simulink model "Test_of_StateFeedbackCtrl_CP_Controller"  (R2023a)
settings: Solver=ode8  StartTime=0.0  StopTime=150  FixedStep=0.001  RelTol=1e-3
libraries: simulink x4
settings Model: Creator=邓宇飞  LastModifiedBy=邓宇飞

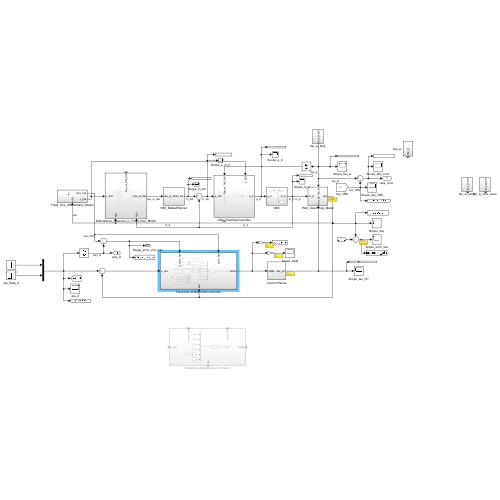
[thumbnail: Simulink's stored preview of the top-level diagram]
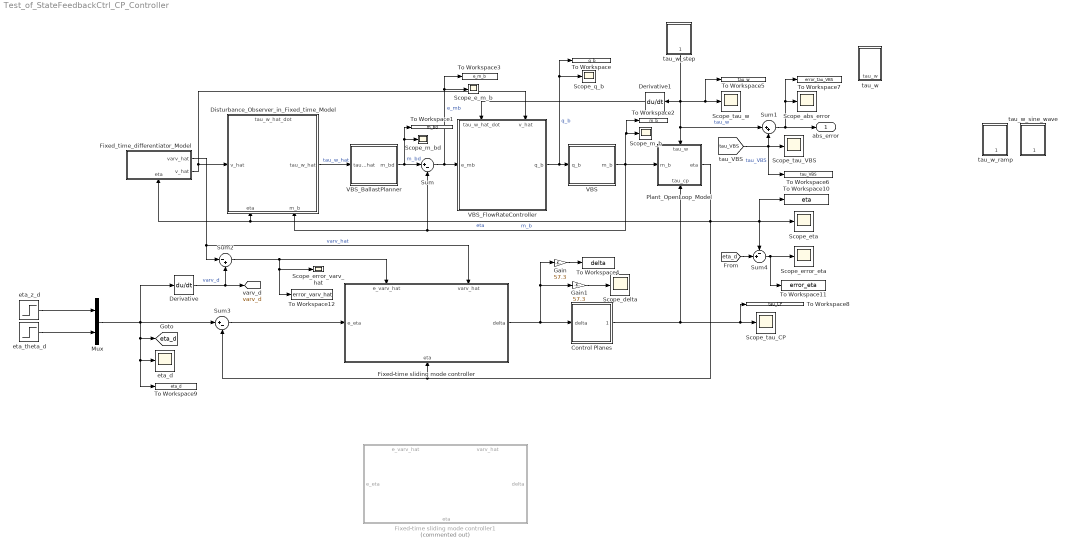
== system Test_of_StateFeedbackCtrl_CP_Controller ==
  Control Planes : Subsystem
  Derivative : Derivative
  Derivative1 : Derivative
  Disturbance_Observer_in_Fixed_time_Model : Subsystem
      settings: PortSchema="{\"entries\":[{\"content\":{\"sides\":[{\"content\":{\"connectorIds\":[\"In1\"]},\"type\":\"ConnectorPlacement.EquallySpacedRectSide\",\"uuid\":\"977a3149-1921-48fe-b96a-a4ad28c91371\"},{\"content\":{\"connectorIds\":[\"Out1\"],\"side\":\"RIGHT\"},\"type\":\"ConnectorPlacement.EquallySpacedRectSide\",\"uuid\":\"fff94096-65c1-4681-8bdf-eed371b61c52\"},{\"content\":{\"connectorIds\":[\"Out2\"],\"side\":\"TOP\"},\"type\":\"ConnectorPlacement.EquallySpacedRectSide\",\"uuid\":\"5bed714d-ab4b-433b-a946-feaea2816cb1\"},{\"content\":{\"connectorIds\":[\"In2\",\"In3\"],\"side\":\"BOTTOM\"},\"type\":\"ConnectorPlacement.EquallySpacedRectSide\",\"uuid\":\"4ad85521-d335-4ab1-88b6-9b8c0a3b2785\"}]},\"type\":\"ConnectorPlacement.EquallySpacedConnector\",\"uuid\":\"7c33b186-f768-465e-b799-f94ef9fdf411\"}],\"packageUris\":[\"http://schema.mathworks.com/mf0/Connector/R2020b\"],\"version\":\"1.0\"}"
  Fixed-time sliding mode controller : Subsystem
      settings: PortSchema="{\"entries\":[{\"content\":{\"sides\":[{\"content\":{\"connectorIds\":[\"In1\"]},\"type\":\"ConnectorPlacement.EquallySpacedRectSide\",\"uuid\":\"f7eec32a-11e5-493e-91a4-aa23e7798835\"},{\"content\":{\"connectorIds\":[\"Out1\"],\"side\":\"RIGHT\"},\"type\":\"ConnectorPlacement.EquallySpacedRectSide\",\"uuid\":\"2b78eec5-73c8-4d02-9319-0fb2d1bcee33\"},{\"content\":{\"connectorIds\":[\"In2\",\"In3\"],\"side\":\"TOP\"},\"type\":\"ConnectorPlacement.EquallySpacedRectSide\",\"uuid\":\"6bb67a89-6549-4a25-872d-286d7aa8440b\"},{\"content\":{\"connectorIds\":[\"In4\"],\"side\":\"BOTTOM\"},\"type\":\"ConnectorPlacement.EquallySpacedRectSide\",\"uuid\":\"a7c480fa-a393-4283-926e-8262b2c36ba1\"}]},\"type\":\"ConnectorPlacement.EquallySpacedConnector\",\"uuid\":\"ac88fafb-ad61-4f2d-a744-8be38b32af3c\"}],\"packageUris\":[\"http://schema.mathworks.com/mf0/Connector/R2020b\"],\"version\":\"1.0\"}"
  Fixed-time sliding mode controller1 : Subsystem  Commented=on
      settings: PortSchema="{\"entries\":[{\"content\":{\"sides\":[{\"content\":{\"connectorIds\":[\"In1\"]},\"type\":\"ConnectorPlacement.EquallySpacedRectSide\",\"uuid\":\"f7eec32a-11e5-493e-91a4-aa23e7798835\"},{\"content\":{\"connectorIds\":[\"Out1\"],\"side\":\"RIGHT\"},\"type\":\"ConnectorPlacement.EquallySpacedRectSide\",\"uuid\":\"2b78eec5-73c8-4d02-9319-0fb2d1bcee33\"},{\"content\":{\"connectorIds\":[\"In2\",\"In3\"],\"side\":\"TOP\"},\"type\":\"ConnectorPlacement.EquallySpacedRectSide\",\"uuid\":\"6bb67a89-6549-4a25-872d-286d7aa8440b\"},{\"content\":{\"connectorIds\":[\"In4\"],\"side\":\"BOTTOM\"},\"type\":\"ConnectorPlacement.EquallySpacedRectSide\",\"uuid\":\"a7c480fa-a393-4283-926e-8262b2c36ba1\"}]},\"type\":\"ConnectorPlacement.EquallySpacedConnector\",\"uuid\":\"ac88fafb-ad61-4f2d-a744-8be38b32af3c\"}],\"packageUris\":[\"http://schema.mathworks.com/mf0/Connector/R2020b\"],\"version\":\"1.0\"}"
  Fixed_time_differentiator_Model : Subsystem
      settings: PortSchema="{\"entries\":[{\"content\":{\"sides\":[{\"content\":{},\"type\":\"ConnectorPlacement.EquallySpacedRectSide\",\"uuid\":\"509b689f-cae1-4523-9372-2499bd3b7d9d\"},{\"content\":{\"connectorIds\":[\"Out1\",\"Out2\"],\"side\":\"RIGHT\"},\"type\":\"ConnectorPlacement.EquallySpacedRectSide\",\"uuid\":\"a1df743b-e6a9-4451-86f2-27990c18dc24\"},{\"content\":{\"side\":\"TOP\"},\"type\":\"ConnectorPlacement.EquallySpacedRectSide\",\"uuid\":\"5149f091-ad88-4d80-a39f-36dd9d24fd7a\"},{\"content\":{\"connectorIds\":[\"In1\"],\"side\":\"BOTTOM\"},\"type\":\"ConnectorPlacement.EquallySpacedRectSide\",\"uuid\":\"b5eefe9f-7883-4d8e-a8af-dce689347657\"}]},\"type\":\"ConnectorPlacement.EquallySpacedConnector\",\"uuid\":\"61175d6f-7ec4-4947-9258-193f13282eb9\"}],\"packageUris\":[\"http://schema.mathworks.com/mf0/Connector/R2020b\"],\"version\":\"1.0\"}"
  Gain : Gain  Gain=57.3
  Gain1 : Gain  Gain=57.3
  Mux : Mux  Inputs=2
  Plant_OpenLoop_Model : Subsystem
      settings: PortSchema="{\"entries\":[{\"content\":{\"sides\":[{\"content\":{\"connectorIds\":[\"In1\"]},\"type\":\"ConnectorPlacement.EquallySpacedRectSide\",\"uuid\":\"171ab365-2c9c-477f-ab94-6e1b535ce398\"},{\"content\":{\"connectorIds\":[\"Out1\"],\"side\":\"RIGHT\"},\"type\":\"ConnectorPlacement.EquallySpacedRectSide\",\"uuid\":\"68d15153-0085-4baf-9515-c294b6b9b8eb\"},{\"content\":{\"connectorIds\":[\"In2\"],\"side\":\"TOP\"},\"type\":\"ConnectorPlacement.EquallySpacedRectSide\",\"uuid\":\"3f887e7e-8b06-4bf2-b39d-d49324deef58\"},{\"content\":{\"connectorIds\":[\"In3\"],\"side\":\"BOTTOM\"},\"type\":\"ConnectorPlacement.EquallySpacedRectSide\",\"uuid\":\"0c56d0aa-527a-42c0-aa98-8ee52c9400f1\"}]},\"type\":\"ConnectorPlacement.EquallySpacedConnector\",\"uuid\":\"a8f2799e-4d6b-4adf-9803-c3f607cd4a91\"}],\"packageUris\":[\"http://schema.mathworks.com/mf0/Connector/R2020b\"],\"version\":\"1.0\"}"
  Scope_abs_error : Scope
  Scope_delta : Scope
  Scope_e_m_b : Scope
  Scope_error_eta : Scope
  Scope_error_varv_hat : Scope
  Scope_eta : Scope
  Scope_m_b : Scope
  Scope_m_bd : Scope
  Scope_q_b : Scope
  Scope_tau_CP : Scope
  Scope_tau_VBS : Scope
  Scope_tau_w : Scope
  Sum : Sum  Inputs=|+-
  Sum1 : Sum  Inputs=|++
  Sum2 : Sum  Inputs=|-+
  Sum3 : Sum  Inputs=|+-
  Sum4 : Sum  Inputs=-+|
  To Workspace : ToWorkspace  VariableName=q_b  SaveFormat=Timeseries  SampleTime=-1
  To Workspace1 : ToWorkspace  VariableName=m_bd  SaveFormat=Timeseries  SampleTime=-1
  To Workspace10 : ToWorkspace  VariableName=eta  SaveFormat=Timeseries  SampleTime=-1
  To Workspace11 : ToWorkspace  VariableName=error_eta  SaveFormat=Timeseries  SampleTime=-1
  To Workspace12 : ToWorkspace  VariableName=error_varv_hat  SaveFormat=Timeseries  SampleTime=-1
  To Workspace2 : ToWorkspace  VariableName=m_b  SaveFormat=Timeseries  SampleTime=-1
  To Workspace3 : ToWorkspace  VariableName=e_m_b  SaveFormat=Timeseries  SampleTime=-1
  To Workspace4 : ToWorkspace  VariableName=delta  SaveFormat=Timeseries  SampleTime=-1
  To Workspace5 : ToWorkspace  VariableName=tau_w  SaveFormat=Timeseries  SampleTime=-1
  To Workspace6 : ToWorkspace  VariableName=tau_VBS  SaveFormat=Timeseries  SampleTime=-1
  To Workspace7 : ToWorkspace  VariableName=error_tau_VBS  SaveFormat=Timeseries  SampleTime=-1
  To Workspace8 : ToWorkspace  VariableName=tau_CP  SaveFormat=Timeseries  SampleTime=-1
  To Workspace9 : ToWorkspace  VariableName=eta_d  SaveFormat=Timeseries  SampleTime=-1
  VBS : Subsystem
  VBS_BallastPlanner : Subsystem
  VBS_FlowRateController : Subsystem
      settings: PortSchema="{\"entries\":[{\"content\":{\"sides\":[{\"content\":{\"connectorIds\":[\"In1\"]},\"type\":\"ConnectorPlacement.EquallySpacedRectSide\",\"uuid\":\"977a3149-1921-48fe-b96a-a4ad28c91371\"},{\"content\":{\"connectorIds\":[\"Out1\"],\"side\":\"RIGHT\"},\"type\":\"ConnectorPlacement.EquallySpacedRectSide\",\"uuid\":\"fff94096-65c1-4681-8bdf-eed371b61c52\"},{\"content\":{\"connectorIds\":[\"In2\",\"In3\"],\"side\":\"TOP\"},\"type\":\"ConnectorPlacement.EquallySpacedRectSide\",\"uuid\":\"5bed714d-ab4b-433b-a946-feaea2816cb1\"}]},\"type\":\"ConnectorPlacement.EquallySpacedConnector\",\"uuid\":\"7c33b186-f768-465e-b799-f94ef9fdf411\"}],\"packageUris\":[\"http://schema.mathworks.com/mf0/Connector/R2020b\"],\"version\":\"1.0\"}"
  eta_d : Scope
  eta_theta_d : Step  Time=0  After=0  SampleTime=0
  eta_z_d : Step  Time=0  Before=1  SampleTime=0
  tau_w : Subsystem
  tau_w_ramp : Subsystem
      settings: PortSchema="{\"entries\":[{\"content\":{\"sides\":[{\"content\":{},\"type\":\"ConnectorPlacement.EquallySpacedRectSide\",\"uuid\":\"4f4de30a-0d0b-4bec-80d6-0206e412bf93\"},{\"content\":{\"side\":\"RIGHT\"},\"type\":\"ConnectorPlacement.EquallySpacedRectSide\",\"uuid\":\"99f054dc-7a49-4f3a-aacd-86d3d985c053\"},{\"content\":{\"side\":\"TOP\"},\"type\":\"ConnectorPlacement.EquallySpacedRectSide\",\"uuid\":\"fb1c8c59-da3b-46d1-8a85-15943150b176\"},{\"content\":{\"connectorIds\":[\"Out1\"],\"side\":\"BOTTOM\"},\"type\":\"ConnectorPlacement.EquallySpacedRectSide\",\"uuid\":\"0ca0dd3c-9837-4edc-a372-abf376ee5c7a\"}]},\"type\":\"ConnectorPlacement.EquallySpacedConnector\",\"uuid\":\"b18296a3-8797-45d2-90ea-b6dd47f9d7d0\"}],\"packageUris\":[\"http://schema.mathworks.com/mf0/Connector/R2020b\"],\"version\":\"1.0\"}"
  tau_w_sine_wave : Subsystem
      settings: PortSchema="{\"entries\":[{\"content\":{\"sides\":[{\"content\":{},\"type\":\"ConnectorPlacement.EquallySpacedRectSide\",\"uuid\":\"4f4de30a-0d0b-4bec-80d6-0206e412bf93\"},{\"content\":{\"side\":\"RIGHT\"},\"type\":\"ConnectorPlacement.EquallySpacedRectSide\",\"uuid\":\"99f054dc-7a49-4f3a-aacd-86d3d985c053\"},{\"content\":{\"side\":\"TOP\"},\"type\":\"ConnectorPlacement.EquallySpacedRectSide\",\"uuid\":\"fb1c8c59-da3b-46d1-8a85-15943150b176\"},{\"content\":{\"connectorIds\":[\"Out1\"],\"side\":\"BOTTOM\"},\"type\":\"ConnectorPlacement.EquallySpacedRectSide\",\"uuid\":\"20ef5005-9f22-4516-b524-19691bb7c6fc\"}]},\"type\":\"ConnectorPlacement.EquallySpacedConnector\",\"uuid\":\"b18296a3-8797-45d2-90ea-b6dd47f9d7d0\"}],\"packageUris\":[\"http://schema.mathworks.com/mf0/Connector/R2020b\"],\"version\":\"1.0\"}"
  tau_w_step : Subsystem
      settings: PortSchema="{\"entries\":[{\"content\":{\"sides\":[{\"content\":{},\"type\":\"ConnectorPlacement.EquallySpacedRectSide\",\"uuid\":\"4f4de30a-0d0b-4bec-80d6-0206e412bf93\"},{\"content\":{\"side\":\"RIGHT\"},\"type\":\"ConnectorPlacement.EquallySpacedRectSide\",\"uuid\":\"99f054dc-7a49-4f3a-aacd-86d3d985c053\"},{\"content\":{\"side\":\"TOP\"},\"type\":\"ConnectorPlacement.EquallySpacedRectSide\",\"uuid\":\"fb1c8c59-da3b-46d1-8a85-15943150b176\"},{\"content\":{\"connectorIds\":[\"Out1\"],\"side\":\"BOTTOM\"},\"type\":\"ConnectorPlacement.EquallySpacedRectSide\",\"uuid\":\"1bc79977-bf79-43c9-a15f-49778b641523\"}]},\"type\":\"ConnectorPlacement.EquallySpacedConnector\",\"uuid\":\"b18296a3-8797-45d2-90ea-b6dd47f9d7d0\"}],\"packageUris\":[\"http://schema.mathworks.com/mf0/Connector/R2020b\"],\"version\":\"1.0\"}"
  abs_error : Outport
  tag scope: eta_d=global, varv_d=global
  wires:
  Fixed-time sliding mode controller/1(delta) -> Gain/1, Gain1/1, Control Planes/1(delta)
  Disturbance_Observer_in_Fixed_time_Model/1(tau_w_hat) -> VBS_BallastPlanner/1(tau_w_hat)  "tau_w_hat"
  VBS_FlowRateController/1(q_b) -> To Workspace/1, Scope_q_b/1, VBS/1(q_b)  "q_b"
  [tau_VBS] -> To Workspace6/1, Scope_tau_VBS/1, Sum1/2  "tau_VBS"
  VBS/1(m_b) -> To Workspace2/1, Scope_m_b/1, Disturbance_Observer_in_Fixed_time_Model/3(m_b), Sum/2, Plant_OpenLoop_Model/1(m_b)  "m_b"
  Plant_OpenLoop_Model/1(eta) -> To Workspace10/1, Sum4/1, Scope_eta/1, Sum3/2, Fixed-time sliding mode controller/4(eta), Fixed_time_differentiator_Model/1(eta), Disturbance_Observer_in_Fixed_time_Model/2(eta)  "eta"
  Sum1/1 -> To Workspace7/1, Scope_abs_error/1, abs_error/1
  tau_w_step/1(tau_w_step) -> Derivative1/1, Plant_OpenLoop_Model/2(tau_w), Sum1/1, To Workspace5/1, Scope_tau_w/1  "tau_w"
  Fixed_time_differentiator_Model/1(varv_hat) -> Fixed-time sliding mode controller/3(varv_hat), Sum2/1  "varv_hat"
  Sum/1 -> VBS_FlowRateController/1(e_mb), To Workspace3/1, Scope_e_m_b/1  "e_mb"
  VBS_BallastPlanner/1(m_bd) -> Sum/1, To Workspace1/1, Scope_m_bd/1  "m_bd"
  Mux/1 -> To Workspace9/1, eta_d/1, [eta_d], Derivative/1, Sum3/1
  Derivative/1 -> [varv_d], Sum2/2  "varv_d"
  Sum2/1 -> Fixed-time sliding mode controller/2(e_varv_hat), To Workspace12/1, Scope_error_varv_hat/1
  Sum3/1 -> Fixed-time sliding mode controller/1(e_eta)
  eta_z_d/1 -> Mux/1
  eta_theta_d/1 -> Mux/2
  Fixed_time_differentiator_Model/2(v_hat) -> Disturbance_Observer_in_Fixed_time_Model/1(v_hat), VBS_FlowRateController/3(v_hat)
  Gain/1 -> To Workspace4/1
  Gain1/1 -> Scope_delta/1
  [eta_d] -> Sum4/2
  Sum4/1 -> To Workspace11/1, Scope_error_eta/1
  Derivative1/1 -> VBS_FlowRateController/2(tau_w_hat_dot)
  Control Planes/1(tau_cp) -> To Workspace8/1, Scope_tau_CP/1, Plant_OpenLoop_Model/3(tau_cp)

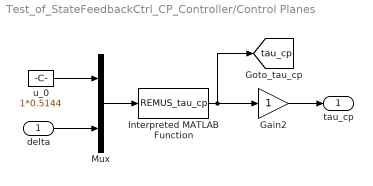
== system Test_of_StateFeedbackCtrl_CP_Controller/Control Planes ==
  delta : Inport
  Gain2 : Gain
  Interpreted MATLAB Function : MATLABFcn  MATLABFcn=REMUS_tau_cp
  Mux : Mux  Inputs=2
  u_0 : Constant  Value=1*0.5144
  tau_cp : Outport
  tag scope: tau_cp=global
  wires:
  delta/1 -> Mux/2
  u_0/1 -> Mux/1
  Mux/1 -> Interpreted MATLAB Function/1
  Interpreted MATLAB Function/1 -> Gain2/1, [tau_cp]
  Gain2/1 -> tau_cp/1

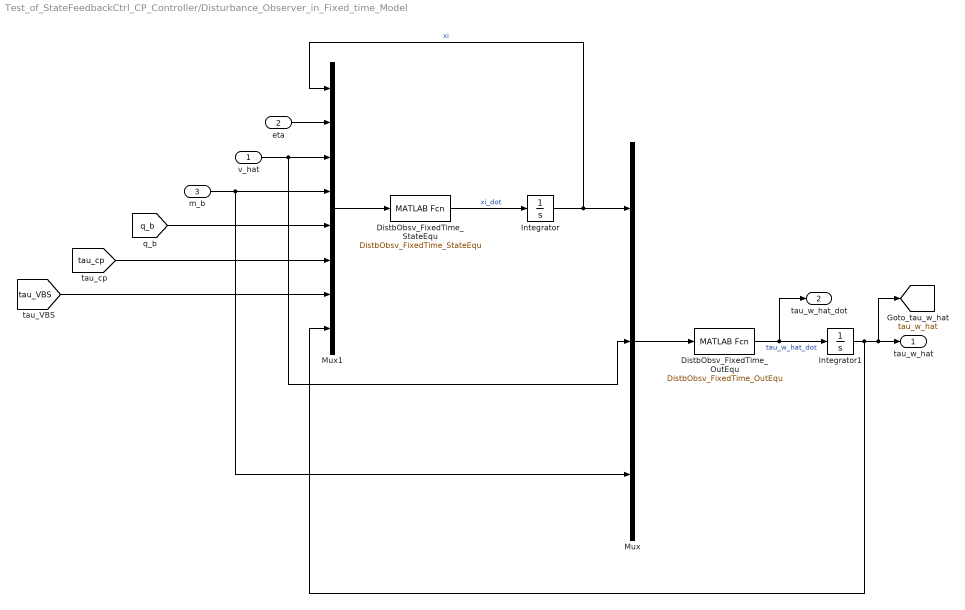
== system Test_of_StateFeedbackCtrl_CP_Controller/Disturbance_Observer_in_Fixed_time_Model ==
  v_hat : Inport
  eta : Inport  Port=2
  m_b : Inport  Port=3
  DistbObsv_FixedTime_OutEqu : MATLABFcn  MATLABFcn=DistbObsv_FixedTime_OutEqu  OutputDimensions=2  OutputSignalType=real
  DistbObsv_FixedTime_StateEqu : MATLABFcn  MATLABFcn=DistbObsv_FixedTime_StateEqu  OutputDimensions=2  OutputSignalType=real
  Integrator : Integrator
  Integrator1 : Integrator
  Mux : Mux  Inputs=3
  Mux1 : Mux  Inputs=8
  tau_w_hat : Outport
  tau_w_hat_dot : Outport  Port=2
  tag scope: tau_w_hat=global
  wires:
  Integrator1/1 -> [tau_w_hat], tau_w_hat/1, Mux1/8
  Integrator/1 -> Mux1/1, Mux/1  "xi"
  DistbObsv_FixedTime_OutEqu/1 -> tau_w_hat_dot/1, Integrator1/1  "tau_w_hat_dot"
  Mux/1 -> DistbObsv_FixedTime_OutEqu/1
  Mux1/1 -> DistbObsv_FixedTime_StateEqu/1
  DistbObsv_FixedTime_StateEqu/1 -> Integrator/1  "xi_dot"
  eta/1 -> Mux1/2
  v_hat/1 -> Mux/2, Mux1/3
  m_b/1 -> Mux/3, Mux1/4
  [q_b] -> Mux1/5
  [tau_cp] -> Mux1/6
  [tau_VBS] -> Mux1/7

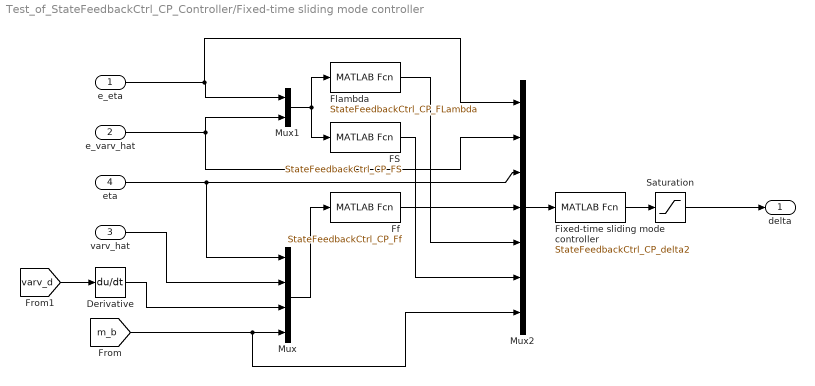
== system Test_of_StateFeedbackCtrl_CP_Controller/Fixed-time sliding mode controller ==
  e_eta : Inport
  e_varv_hat : Inport  Port=2
  varv_hat : Inport  Port=3
  eta : Inport  Port=4
  Derivative : Derivative
  FS : MATLABFcn  MATLABFcn=StateFeedbackCtrl_CP_FS  OutputDimensions=2  OutputSignalType=real
  Ff : MATLABFcn  MATLABFcn=StateFeedbackCtrl_CP_Ff  OutputDimensions=2  OutputSignalType=real
  Fixed-time sliding mode controller : MATLABFcn  MATLABFcn=StateFeedbackCtrl_CP_delta2  OutputDimensions=2  OutputSignalType=real
  Flambda : MATLABFcn  MATLABFcn=StateFeedbackCtrl_CP_FLambda  OutputDimensions=2  OutputSignalType=real
  Mux : Mux
  Mux1 : Mux  Inputs=2
  Mux2 : Mux  Inputs=7
  Saturation : Saturate  UpperLimit=pi/6  LowerLimit=-pi/6
  delta : Outport
  wires:
  eta/1 -> Mux2/3, Mux/1
  Derivative/1 -> Mux/3
  varv_hat/1 -> Mux/2
  e_eta/1 -> Mux2/1, Mux1/1
  e_varv_hat/1 -> Mux1/2, Mux2/2
  Fixed-time sliding mode controller/1 -> Saturation/1
  [varv_d] -> Derivative/1
  Mux/1 -> Ff/1
  [m_b] -> Mux2/7, Mux/4
  Mux1/1 -> Flambda/1, FS/1
  Ff/1 -> Mux2/4
  Flambda/1 -> Mux2/5
  FS/1 -> Mux2/6
  Mux2/1 -> Fixed-time sliding mode controller/1
  Saturation/1 -> delta/1

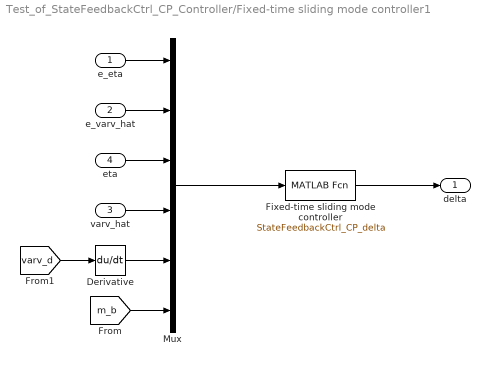
== system Test_of_StateFeedbackCtrl_CP_Controller/Fixed-time sliding mode controller1 ==
  e_eta : Inport
  e_varv_hat : Inport  Port=2
  varv_hat : Inport  Port=3
  eta : Inport  Port=4
  Derivative : Derivative
  Fixed-time sliding mode controller : MATLABFcn  MATLABFcn=StateFeedbackCtrl_CP_delta  OutputDimensions=2  OutputSignalType=real
  Mux : Mux  Inputs=6
  delta : Outport
  wires:
  eta/1 -> Mux/3
  Derivative/1 -> Mux/5
  varv_hat/1 -> Mux/4
  [m_b] -> Mux/6
  e_eta/1 -> Mux/1
  Mux/1 -> Fixed-time sliding mode controller/1
  e_varv_hat/1 -> Mux/2
  Fixed-time sliding mode controller/1 -> delta/1
  [varv_d] -> Derivative/1

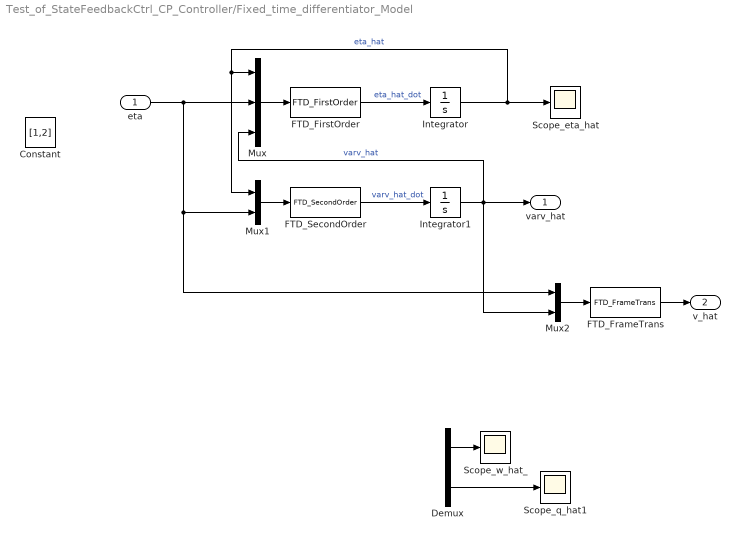
== system Test_of_StateFeedbackCtrl_CP_Controller/Fixed_time_differentiator_Model ==
  eta : Inport
  Constant : Constant  Value=[1,2]
  Demux : Demux  Outputs=2
  FTD_FirstOrder : MATLABFcn  MATLABFcn=FTD_FirstOrder  OutputDimensions=2
  FTD_FrameTrans : MATLABFcn  MATLABFcn=FTD_FrameTrans
  FTD_SecondOrder : MATLABFcn  MATLABFcn=FTD_SecondOrder  OutputDimensions=2
  Integrator : Integrator
  Integrator1 : Integrator
  Mux : Mux  Inputs=3
  Mux1 : Mux  Inputs=2
  Mux2 : Mux  Inputs=2
  Scope_eta_hat : Scope
  Scope_q_hat1 : Scope
  Scope_w_hat_ : Scope
  varv_hat : Outport
  v_hat : Outport  Port=2
  wires:
  Demux/1 -> Scope_w_hat_/1
  Integrator/1 -> Mux1/1, Mux/1, Scope_eta_hat/1  "eta_hat"
  Integrator1/1 -> Mux2/2, varv_hat/1, Mux/3  "varv_hat"
  Mux/1 -> FTD_FirstOrder/1
  Mux1/1 -> FTD_SecondOrder/1
  Demux/2 -> Scope_q_hat1/1
  FTD_SecondOrder/1 -> Integrator1/1  "varv_hat_dot"
  FTD_FirstOrder/1 -> Integrator/1  "eta_hat_dot"
  FTD_FrameTrans/1 -> v_hat/1
  Mux2/1 -> FTD_FrameTrans/1
  eta/1 -> Mux2/1, Mux1/2, Mux/2

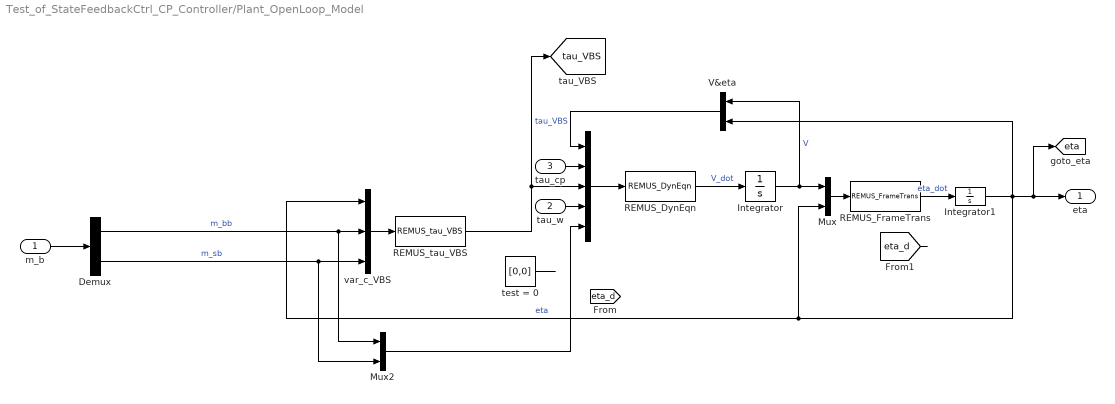
== system Test_of_StateFeedbackCtrl_CP_Controller/Plant_OpenLoop_Model ==
  m_b : Inport
  tau_w : Inport  Port=2
  tau_cp : Inport  Port=3
  " " : Mux  Inputs=5
  Demux : Demux  Outputs=2
  Integrator : Integrator
  Integrator1 : Integrator  InitialCondition=[0;0]
  Mux : Mux  Inputs=2
  Mux2 : Mux  Inputs=2
  REMUS_DynEqn : MATLABFcn  MATLABFcn=REMUS_DynEqn  OutputDimensions=2
  REMUS_FrameTrans : MATLABFcn  MATLABFcn=REMUS_FrameTrans  OutputDimensions=2
  REMUS_tau_VBS : MATLABFcn  MATLABFcn=REMUS_tau_VBS  OutputDimensions=2
  V&eta : Mux  Inputs=2
  test = 0 : Constant  Value=[0,0]
  var_c_VBS : Mux  Inputs=3
  eta : Outport
  tag scope: eta=global, tau_VBS=global
  wires:
  REMUS_DynEqn/1 -> Integrator/1  "V_dot"
  Integrator1/1 -> Mux/2, var_c_VBS/1, [eta], eta/1, V&eta/2  "eta"
  test = 0/1 -> ?
  Demux/2 -> Mux2/2, var_c_VBS/3  "m_sb"
  Mux/1 -> REMUS_FrameTrans/1
  " "/1 -> REMUS_DynEqn/1
  Integrator/1 -> Mux/1, V&eta/1  "V"
  Demux/1 -> Mux2/1, var_c_VBS/2  "m_bb"
  V&eta/1 -> " "/1
  REMUS_tau_VBS/1 -> [tau_VBS], " "/3  "tau_VBS"
  tau_w/1 -> " "/4
  REMUS_FrameTrans/1 -> Integrator1/1  "eta_dot"
  var_c_VBS/1 -> REMUS_tau_VBS/1
  Mux2/1 -> " "/5
  m_b/1 -> Demux/1
  tau_cp/1 -> " "/2
  [eta_d] -> ?

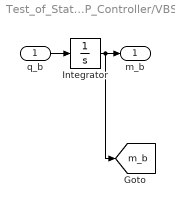
== system Test_of_StateFeedbackCtrl_CP_Controller/VBS ==
  q_b : Inport
  Integrator : Integrator
  m_b : Outport
  tag scope: m_b=global
  wires:
  q_b/1 -> Integrator/1
  Integrator/1 -> [m_b], m_b/1

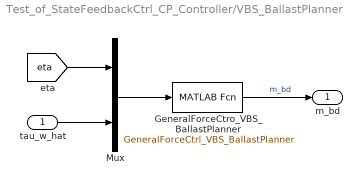
== system Test_of_StateFeedbackCtrl_CP_Controller/VBS_BallastPlanner ==
  tau_w_hat : Inport
  GeneralForceCtro_VBS_BallastPlanner : MATLABFcn  MATLABFcn=GeneralForceCtrl_VBS_BallastPlanner  OutputDimensions=2  OutputSignalType=real
  Mux : Mux  Inputs=2
  m_bd : Outport
  wires:
  Mux/1 -> GeneralForceCtro_VBS_BallastPlanner/1
  GeneralForceCtro_VBS_BallastPlanner/1 -> m_bd/1  "m_bd"
  [eta] -> Mux/1
  tau_w_hat/1 -> Mux/2

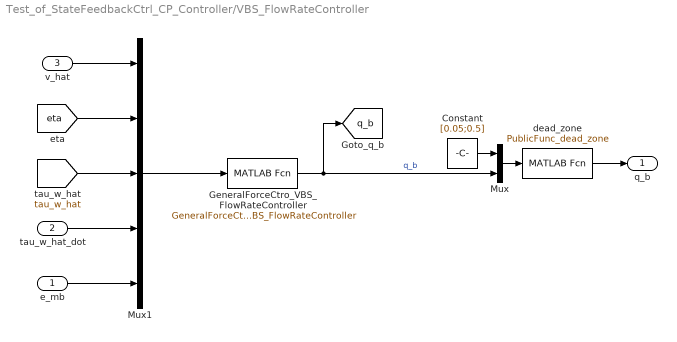
== system Test_of_StateFeedbackCtrl_CP_Controller/VBS_FlowRateController ==
  e_mb : Inport
  tau_w_hat_dot : Inport  Port=2
  v_hat : Inport  Port=3
  Constant : Constant  Value=[0.05;0.5]
  GeneralForceCtro_VBS_FlowRateController : MATLABFcn  MATLABFcn=GeneralForceCtrl_VBS_FlowRateController  OutputDimensions=2  OutputSignalType=real
  Mux : Mux  Inputs=2
  Mux1 : Mux  Inputs=5
  dead_zone : MATLABFcn  MATLABFcn=PublicFunc_dead_zone
  q_b : Outport
  tag scope: q_b=global
  wires:
  Mux1/1 -> GeneralForceCtro_VBS_FlowRateController/1
  GeneralForceCtro_VBS_FlowRateController/1 -> Mux/2, [q_b]  "q_b"
  v_hat/1 -> Mux1/1
  [eta] -> Mux1/2
  [tau_w_hat] -> Mux1/3
  tau_w_hat_dot/1 -> Mux1/4
  e_mb/1 -> Mux1/5
  dead_zone/1 -> q_b/1
  Constant/1 -> Mux/1
  Mux/1 -> dead_zone/1

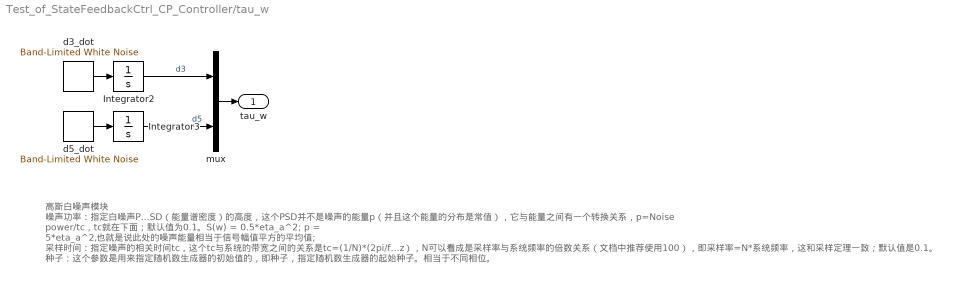
== system Test_of_StateFeedbackCtrl_CP_Controller/tau_w ==
  note: 高斯白噪声模块
      | 噪声功率：指定白噪声PSD（能量谱密度）的高度，这个PSD并不是噪声的能量p（并且这个能量的分布是常值），它与能量之间有一个转换关系，p=Noise power/tc，tc就在下面；默认值为0.1。S(w) = 0.5*eta_a^2;
      | p = 5*eta_a^2;也就是说此处的噪声能量相当于信号幅值平方的平均值;
      | 采样时间：指定噪声的相关时间tc，这个tc与系统的带宽之间的关系是tc=(1/N)*(2pi/fmax)，其中fmax是系统的带宽（实际上是角频率，fmax=2*pi*f，这个f才是我们常使用的频率Hz），N可以看成是采样率与系统频率的倍数关系（文档中推荐使用100），即采样率=N*系统频率，这和采样定理一致；默认值是0.1。
      | 种子：这个参数是用来指定随机数生成器的初始值的，即种子，指定随机数生成器的起始种子。相当于不同相位。
  Integrator2 : Integrator
  Integrator3 : Integrator
  d3_dot : simulink/Sources/Band-Limited White Noise  Cov=[0.5]  Ts=0.1  seed=[2]
  d5_dot : simulink/Sources/Band-Limited White Noise  Cov=[0.1]  Ts=0.1  seed=[3]
  mux : Mux  Inputs=2
  tau_w : Outport
  wires:
  Integrator3/1 -> mux/2  "d5"
  d5_dot/1 -> Integrator3/1
  d3_dot/1 -> Integrator2/1
  mux/1 -> tau_w/1
  Integrator2/1 -> mux/1  "d3"

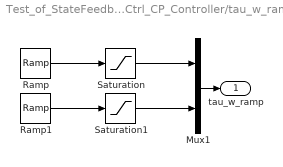
== system Test_of_StateFeedbackCtrl_CP_Controller/tau_w_ramp ==
  Mux1 : Mux  Inputs=2
  Ramp : simulink/Sources/Ramp  slope=1  start=0  InitialOutput=0
  Ramp1 : simulink/Sources/Ramp  slope=1  start=0  InitialOutput=0
  Saturation : Saturate  UpperLimit=10  LowerLimit=0
  Saturation1 : Saturate  UpperLimit=10  LowerLimit=0
  tau_w_ramp : Outport
  wires:
  Mux1/1 -> tau_w_ramp/1
  Ramp/1 -> Saturation/1
  Saturation/1 -> Mux1/1
  Ramp1/1 -> Saturation1/1
  Saturation1/1 -> Mux1/2

== system Test_of_StateFeedbackCtrl_CP_Controller/tau_w_sine_wave ==
  Mux2 : Mux  Inputs=2
  Sine Wave : Sin  Amplitude=15  Frequency=0.1*pi  Phase=0.5*pi  SampleTime=0
  Sine Wave1 : Sin  Amplitude=15  Frequency=0.1*pi  Phase=0.5*pi  SampleTime=0
  tau_w_sine_wave : Outport
  wires:
  Sine Wave1/1 -> Mux2/2
  Sine Wave/1 -> Mux2/1
  Mux2/1 -> tau_w_sine_wave/1

== system Test_of_StateFeedbackCtrl_CP_Controller/tau_w_step ==
  Mux : Mux  Inputs=2
  Step : Step  After=0  SampleTime=0
  Step1 : Step  After=0  SampleTime=0
  tau_w_step : Outport
  wires:
  Step1/1 -> Mux/2
  Step/1 -> Mux/1
  Mux/1 -> tau_w_step/1
